simulink model "Lab1_5"  (R2018a)
settings: Solver=VariableStepAuto  StartTime=0.0  StopTime=10.0  RelTol=1e-3
settings Model: Creator=rahul  LastModifiedBy=melab2
settings CodeAppCC: StateflowObjectComments=on

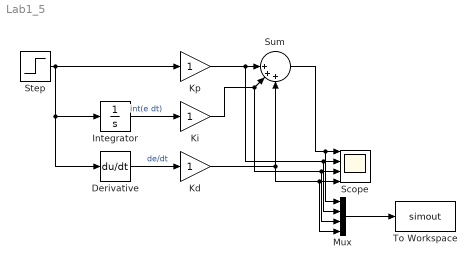
== system Lab1_5 ==
  Derivative : Derivative
  Integrator : Integrator
  Kd : Gain
  Ki : Gain
  Kp : Gain
  Mux : Mux
  Scope : Scope  NumInputPorts=4
  Step : Step  SampleTime=0
  Sum : Sum  Inputs=||+++
  To Workspace : ToWorkspace  VariableName=simout  SampleTime=-1
  wires:
  Integrator/1 -> Ki/1  "int(e dt)"
  Derivative/1 -> Kd/1  "de/dt"
  Kp/1 -> Mux/2, Scope/2, Sum/1
  Ki/1 -> Mux/3, Scope/3, Sum/2
  Kd/1 -> Mux/4, Scope/4, Sum/3
  Sum/1 -> Mux/1, Scope/1
  Step/1 -> Derivative/1, Integrator/1, Kp/1
  Mux/1 -> To Workspace/1
